simulink model "Steering_Controller"  (R2018b)
settings: Solver=FixedStepDiscrete  StartTime=0.0  StopTime=10.0  FixedStep=Step_Size  RelTol=1e-3
values from neighbouring files (symbols this model uses):
  Encoder_Counts_Per_Degree = Simulink.Parameter    [init.m]    (also in init_shared_parameters.m)
  Kd = 0    [init.m]    (also in init_Steering_Controller.m)
  Kp = 10.0    (= 10)    [init.m]    (also in init_Steering_Controller.m)
  Power_Level_Max = 100    [init.m]    (also in init_Steering_Controller.m)
  Power_Level_Min = -100    [init.m]    (also in init_Steering_Controller.m)
  Steering_Offset = Simulink.Parameter    [init.m]    (also in init_NXT_Motor.m; init_Steering_Controller.m; init_Steering_Subsystem.m = 45)
  To_The_Left = Simulink.Parameter    [init.m]    (also in init_shared_parameters.m)
  To_The_Right = Simulink.Parameter    [init.m]    (also in init_shared_parameters.m)
undefined symbols (not defined in the file or in its folder): DiscIntNeverNeededParam
settings Model: Creator=tony  LastModifiedBy=tony
settings OptimizationCC: BlockReduction=off
settings DebuggingCC: ConsistencyChecking=error  SignalInfNanChecking=error  SignalRangeChecking=error  AlgebraicLoopMsg=error  SigSpecEnsureSampleTimeMsg=error  IntegerOverflowMsg=error  ParameterUnderflowMsg=error  ParameterPrecisionLossMsg=error  ParameterTunabilityLossMsg=error  SFcnCompatibilityMsg=error  BusObjectLabelMismatch=error  RootOutportRequireBusObject=error  AllowSymbolicDim=off  ModelReferenceVersionMismatchMessage=error  ModelReferenceIOMismatchMessage=error  UnknownTsInhSupMsg=error  StrictBusMsg=ErrorOnBusTreatedAsVector  BusNameAdapt=ErrorWithoutRepair  NonBusSignalsTreatedAsBus=error  SFInvalidInputDataAccessInChartInitDiag=error  SFTransitionOutsideNaturalParentDiag=error  SFUnreachableExecutionPathDiag=error  SFExecutionAtInitializationDiag=error  SFMachineParentedDataDiag=error  IntegerSaturationMsg=error  AllowAutomaticUnitConversions=off
settings SFSimCC: SimUseLocalCustomCode=off  SimParseCustomCode=off

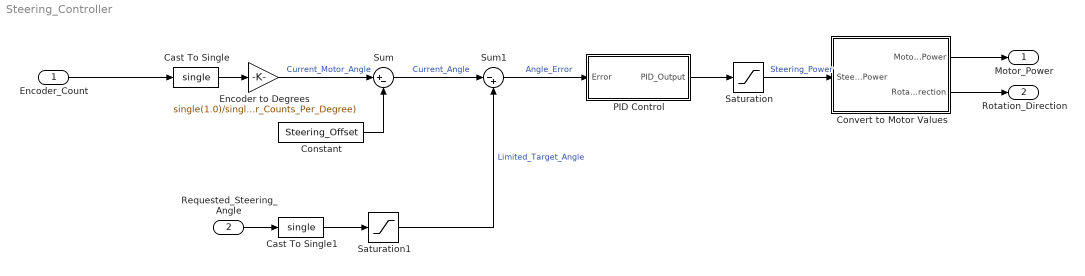
== system Steering_Controller ==
  Encoder_Count : Inport  OutDataTypeStr=Motor_Encoder_Counts
  Requested_Steering_Angle : Inport  Port=2  OutDataTypeStr=int8
  Cast To Single : DataTypeConversion  OutDataTypeStr=single
  Cast To Single1 : DataTypeConversion  OutDataTypeStr=single
  Constant : Constant  Value=Steering_Offset
  Convert to Motor Values : Subsystem
  Encoder to Degrees : Gain  Gain=single(1.0)/single(Encoder_Counts_Per_Degree)  ParamDataTypeStr=single  RndMeth=Zero  OutDataTypeStr=Inherit: Same as input
  PID Control : Subsystem
  Saturation : Saturate  UpperLimit=Power_Level_Max  LowerLimit=Power_Level_Min
  Saturation1 : Saturate  UpperLimit=Steering_Offset  LowerLimit=-Steering_Offset
  Sum : Sum  Inputs=|+-
  Sum1 : Sum  Inputs=|-+
  Motor_Power : Outport
  Rotation_Direction : Outport  Port=2
  wires:
  PID Control/1(PID_Output) -> Saturation/1
  Requested_Steering_Angle/1 -> Cast To Single1/1
  Constant/1 -> Sum/2
  Encoder to Degrees/1 -> Sum/1  "Current_Motor_Angle"
  Sum/1 -> Sum1/1  "Current_Angle"
  Saturation1/1 -> Sum1/2  "Limited_Target_Angle"
  Sum1/1 -> PID Control/1(Error)  "Angle_Error"
  Saturation/1 -> Convert to Motor Values/1(Steering_Power)  "Steering_Power"
  Encoder_Count/1 -> Cast To Single/1
  Convert to Motor Values/2(Rotation_Direction) -> Rotation_Direction/1
  Convert to Motor Values/1(Motor_Power) -> Motor_Power/1
  Cast To Single/1 -> Encoder to Degrees/1
  Cast To Single1/1 -> Saturation1/1

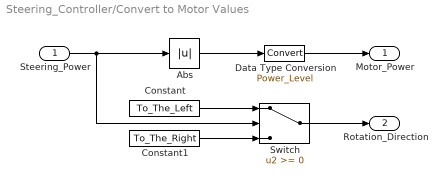
== system Steering_Controller/Convert to Motor Values ==
  Steering_Power : Inport
  Abs : Abs
  Constant : Constant  Value=To_The_Left
  Constant1 : Constant  Value=To_The_Right
  Data Type Conversion : DataTypeConversion  OutDataTypeStr=Power_Level  RndMeth=Zero
  Switch : Switch
  Motor_Power : Outport
  Rotation_Direction : Outport  Port=2
  wires:
  Steering_Power/1 -> Abs/1, Switch/2
  Abs/1 -> Data Type Conversion/1
  Switch/1 -> Rotation_Direction/1
  Constant/1 -> Switch/1
  Constant1/1 -> Switch/3
  Data Type Conversion/1 -> Motor_Power/1

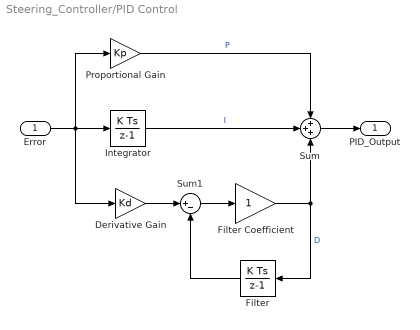
== system Steering_Controller/PID Control ==
  Error : Inport
  Derivative Gain : Gain  Gain=Kd
  Filter : DiscreteIntegrator  gainval=1  SampleTime=-1  ICPrevOutput=DiscIntNeverNeededParam  ICPrevScaledInput=DiscIntNeverNeededParam
  Filter Coefficient : Gain
  Integrator : DiscreteIntegrator  gainval=Ki  SampleTime=-1  ICPrevOutput=DiscIntNeverNeededParam  ICPrevScaledInput=DiscIntNeverNeededParam
  Proportional Gain : Gain  Gain=Kp
  Sum : Sum  Inputs=+++
  Sum1 : Sum  Inputs=|+-
  PID_Output : Outport
  wires:
  Derivative Gain/1 -> Sum1/1
  Sum1/1 -> Filter Coefficient/1
  Filter/1 -> Sum1/2
  Filter Coefficient/1 -> Filter/1, Sum/3  "D"
  Integrator/1 -> Sum/2  "I"
  Proportional Gain/1 -> Sum/1  "P"
  Error/1 -> Derivative Gain/1, Proportional Gain/1, Integrator/1
  Sum/1 -> PID_Output/1
